simulink model "chp92simulation"  (R2019a)
settings: Solver=VariableStepAuto  StartTime=0.0  StopTime=10.0  RelTol=1e-3
settings Model: Creator=zkibria  LastModifiedBy=zkibria

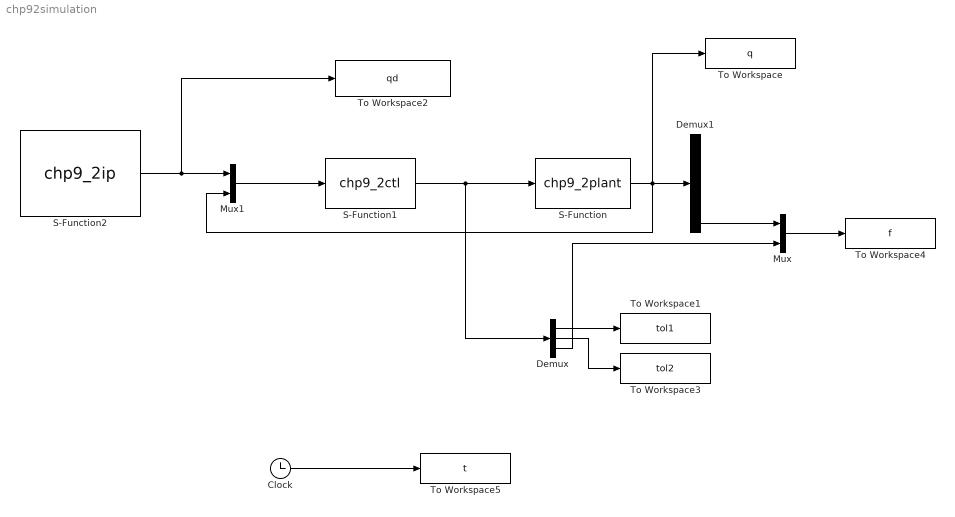
== system chp92simulation ==
  Clock : Clock
  Demux : Demux  Outputs=3
  Demux1 : Demux  Outputs=5
  Mux : Mux  Inputs=2
  Mux1 : Mux  Inputs=2
  S-Function : S-Function  FunctionName=chp9_2plant  SFunctionDeploymentMode=off  EnableBusSupport=off
  S-Function1 : S-Function  FunctionName=chp9_2ctl  SFunctionDeploymentMode=off  EnableBusSupport=off
  S-Function2 : S-Function  FunctionName=chp9_2ip  SFunctionDeploymentMode=off  EnableBusSupport=off
  To Workspace : ToWorkspace  VariableName=q  SaveFormat=Timeseries  SampleTime=-1
  To Workspace1 : ToWorkspace  VariableName=tol1  SaveFormat=Timeseries  SampleTime=-1
  To Workspace2 : ToWorkspace  VariableName=qd  SaveFormat=Timeseries  SampleTime=-1
  To Workspace3 : ToWorkspace  VariableName=tol2  SaveFormat=Timeseries  SampleTime=-1
  To Workspace4 : ToWorkspace  VariableName=f  SaveFormat=Timeseries  SampleTime=-1
  To Workspace5 : ToWorkspace  VariableName=t  SaveFormat=Timeseries  SampleTime=-1
  wires:
  Clock/1 -> To Workspace5/1
  S-Function2/1 -> To Workspace2/1, Mux1/1
  Mux1/1 -> S-Function1/1
  S-Function1/1 -> Demux/1, S-Function/1
  S-Function/1 -> To Workspace/1, Mux1/2, Demux1/1
  Demux1/5 -> Mux/1
  Demux/1 -> To Workspace1/1
  Demux/2 -> To Workspace3/1
  Demux/3 -> Mux/2
  Mux/1 -> To Workspace4/1
